simulink model "bbw"  (Simulink 8.7)
settings: Solver=FixedStepDiscrete  StartTime=0.0  StopTime=30  FixedStep=T_sim  RelTol=1e-6
PostLoadFcn:
  | parameters
undefined symbols (not defined in the file): distrib, Fc_table_x, Fc_table_y, I, M, maxBrakeTorque, R, slip_abs_on, T_abs, T_brake_ctrl, T_brake_pedal, T_spd_est, T_veh, use_division, v0, v_max, w0, w_max
settings Model: Creator=yt59680  LastModifiedBy=pfj01
settings SolverCC: AutoInsertRateTranBlk=on
settings DataIOCC: SignalLoggingSaveFormat=ModelDataLogs
settings OptimizationCC: ExpressionDepthLimit=2147483647
settings DebuggingCC: SolverPrmCheckMsg=warning  InvalidFcnCallConnMsg=warning  FcnCallInpInsideContextMsg=UseLocalSettings  AllowSymbolicDim=off  StateNameClashWarn=warning  StrictBusMsg=Warning
settings HardwareCC: TargetBitPerPointer=64  TargetLongLongMode=on  TargetIntDivRoundTo=Zero  TargetEndianess=LittleEndian  TargetWordSize=64  TargetHWDeviceType=MATLAB Host  ProdEqTarget=off
settings RTWCC: SystemTargetFile=rsim.tlc  TemplateMakefile=rsim_default_tmf  Description=Rapid Simulation Target
settings TargetCC: ParMdlRefBuildCompliant=on  ConcurrentExecutionCompliant=on  MatFileLogging=on
settings CustomProperty: DataType=string  Value=Auto

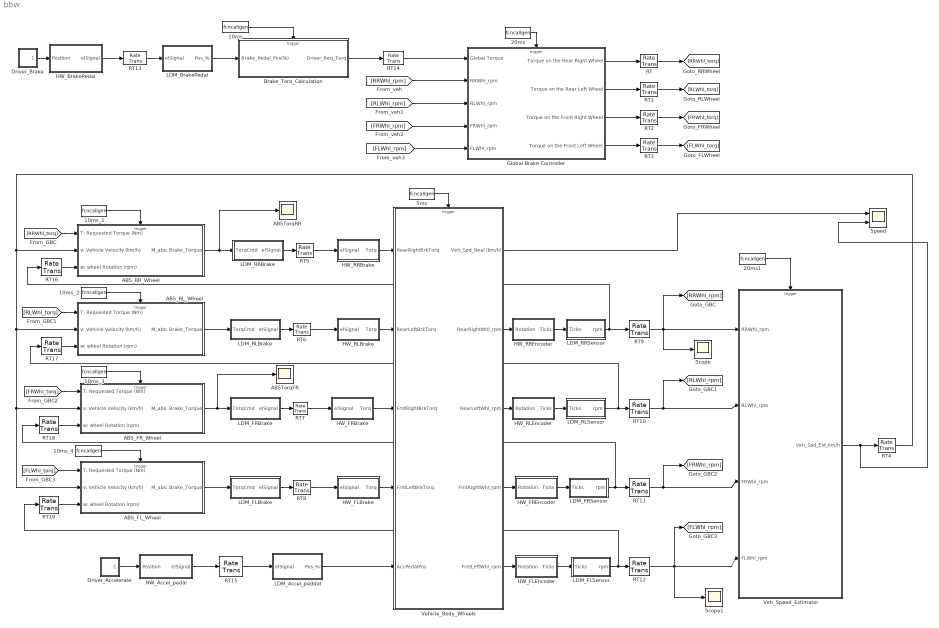
== system bbw ==
  10ms : S-Function  FunctionName=fcncallgen  Parameters=sample_time,numberOfIterations  SFunctionDeploymentMode=off  EnableBusSupport=off  mask(Function-Call Generator){sample_time=T_brake_pedal, numberOfIterations=1}
      mask prompts: sample_time "Simulink:masks:SampleTime_MP"; numberOfIterations "Simulink:masks:NumberOfIterations_MP"
      mask help: Simulink:masks:FunctionCallGenerator_MD
      mask init:
      | if ~isempty(numberOfIterations) & length(numberOfIterations) == 1 & (numberOfIterations > 1),
      | str=sprintf('iterate I = 1:%d',numberOfIterations);
      | else, str = 'f()';
      | end;
      mask Help: This block executes a function-call subsystem at the rate specified by the sample time and a specified number of times.
      mask Display: disp(str)
  10ms_1 : S-Function  FunctionName=fcncallgen  Parameters=sample_time,numberOfIterations  SFunctionDeploymentMode=off  EnableBusSupport=off  mask(Function-Call Generator){sample_time=T_abs, numberOfIterations=1}
      mask prompts: sample_time "Simulink:masks:SampleTime_MP"; numberOfIterations "Simulink:masks:NumberOfIterations_MP"
      mask help: Simulink:masks:FunctionCallGenerator_MD
      mask init:
      | if ~isempty(numberOfIterations) & length(numberOfIterations) == 1 & (numberOfIterations > 1),
      | str=sprintf('iterate I = 1:%d',numberOfIterations);
      | else, str = 'f()';
      | end;
      mask Help: This block executes a function-call subsystem at the rate specified by the sample time and a specified number of times.
      mask Display: disp(str)
  10ms_2 : S-Function  FunctionName=fcncallgen  Parameters=sample_time,numberOfIterations  SFunctionDeploymentMode=off  EnableBusSupport=off  mask(Function-Call Generator){sample_time=T_abs, numberOfIterations=1}
      mask prompts: sample_time "Simulink:masks:SampleTime_MP"; numberOfIterations "Simulink:masks:NumberOfIterations_MP"
      mask help: Simulink:masks:FunctionCallGenerator_MD
      mask init:
      | if ~isempty(numberOfIterations) & length(numberOfIterations) == 1 & (numberOfIterations > 1),
      | str=sprintf('iterate I = 1:%d',numberOfIterations);
      | else, str = 'f()';
      | end;
      mask Help: This block executes a function-call subsystem at the rate specified by the sample time and a specified number of times.
      mask Display: disp(str)
  10ms_3 : S-Function  FunctionName=fcncallgen  Parameters=sample_time,numberOfIterations  SFunctionDeploymentMode=off  EnableBusSupport=off  mask(Function-Call Generator){sample_time=T_abs, numberOfIterations=1}
      mask prompts: sample_time "Simulink:masks:SampleTime_MP"; numberOfIterations "Simulink:masks:NumberOfIterations_MP"
      mask help: Simulink:masks:FunctionCallGenerator_MD
      mask init:
      | if ~isempty(numberOfIterations) & length(numberOfIterations) == 1 & (numberOfIterations > 1),
      | str=sprintf('iterate I = 1:%d',numberOfIterations);
      | else, str = 'f()';
      | end;
      mask Help: This block executes a function-call subsystem at the rate specified by the sample time and a specified number of times.
      mask Display: disp(str)
  10ms_4 : S-Function  FunctionName=fcncallgen  Parameters=sample_time,numberOfIterations  SFunctionDeploymentMode=off  EnableBusSupport=off  mask(Function-Call Generator){sample_time=T_abs, numberOfIterations=1}
      mask prompts: sample_time "Simulink:masks:SampleTime_MP"; numberOfIterations "Simulink:masks:NumberOfIterations_MP"
      mask help: Simulink:masks:FunctionCallGenerator_MD
      mask init:
      | if ~isempty(numberOfIterations) & length(numberOfIterations) == 1 & (numberOfIterations > 1),
      | str=sprintf('iterate I = 1:%d',numberOfIterations);
      | else, str = 'f()';
      | end;
      mask Help: This block executes a function-call subsystem at the rate specified by the sample time and a specified number of times.
      mask Display: disp(str)
  20ms : S-Function  FunctionName=fcncallgen  Parameters=sample_time,numberOfIterations  SFunctionDeploymentMode=off  EnableBusSupport=off  mask(Function-Call Generator){sample_time=T_brake_ctrl, numberOfIterations=1}
      mask prompts: sample_time "Simulink:masks:SampleTime_MP"; numberOfIterations "Simulink:masks:NumberOfIterations_MP"
      mask help: Simulink:masks:FunctionCallGenerator_MD
      mask init:
      | if ~isempty(numberOfIterations) & length(numberOfIterations) == 1 & (numberOfIterations > 1),
      | str=sprintf('iterate I = 1:%d',numberOfIterations);
      | else, str = 'f()';
      | end;
      mask Help: This block executes a function-call subsystem at the rate specified by the sample time and a specified number of times.
      mask Display: disp(str)
  20ms1 : S-Function  FunctionName=fcncallgen  Parameters=sample_time,numberOfIterations  SFunctionDeploymentMode=off  EnableBusSupport=off  mask(Function-Call Generator){sample_time=T_spd_est, numberOfIterations=1}
      mask prompts: sample_time "Simulink:masks:SampleTime_MP"; numberOfIterations "Simulink:masks:NumberOfIterations_MP"
      mask help: Simulink:masks:FunctionCallGenerator_MD
      mask init:
      | if ~isempty(numberOfIterations) & length(numberOfIterations) == 1 & (numberOfIterations > 1),
      | str=sprintf('iterate I = 1:%d',numberOfIterations);
      | else, str = 'f()';
      | end;
      mask Help: This block executes a function-call subsystem at the rate specified by the sample time and a specified number of times.
      mask Display: disp(str)
  5ms : S-Function  FunctionName=fcncallgen  Parameters=sample_time,numberOfIterations  SFunctionDeploymentMode=off  EnableBusSupport=off  mask(Function-Call Generator){sample_time=T_veh, numberOfIterations=1}
      mask prompts: sample_time "Simulink:masks:SampleTime_MP"; numberOfIterations "Simulink:masks:NumberOfIterations_MP"
      mask help: Simulink:masks:FunctionCallGenerator_MD
      mask init:
      | if ~isempty(numberOfIterations) & length(numberOfIterations) == 1 & (numberOfIterations > 1),
      | str=sprintf('iterate I = 1:%d',numberOfIterations);
      | else, str = 'f()';
      | end;
      mask Help: This block executes a function-call subsystem at the rate specified by the sample time and a specified number of times.
      mask Display: disp(str)
  ABSTorqFR : Scope
  ABSTorqRR : Scope
  ABS_FL_Wheel : Subsystem  TreatAsAtomicUnit=on
  ABS_FR_Wheel : Subsystem  TreatAsAtomicUnit=on
  ABS_RL_Wheel : Subsystem  TreatAsAtomicUnit=on
  ABS_RR_Wheel : Subsystem  TreatAsAtomicUnit=on
  Brake_Torq_Calculation : Subsystem  TreatAsAtomicUnit=on
  Driver_Accelerate : Subsystem  mask(Repeating table){rep_seq_t=[0 1 10.5 11 100], rep_seq_y=[0 100 100 0 0]}
      mask prompts: rep_seq_t "Simulink:masks:TimeValues_MP"; rep_seq_y "Simulink:masks:OutputValues_MP"
      mask help: Simulink:masks:RepeatingTable_MD
      mask init:
      | X = [];
      | Y = [];
      | if (length(rep_seq_t) ~= length(rep_seq_y)),
      |   error('Length of time vector and output vector must be the same.')
      | end
      | dbl_rep_seq_t = double(rep_seq_t);
      | dbl_rep_seq_y = double(rep_seq_y);
      | period = max(dbl_rep_seq_t) - min(dbl_rep_seq_t);
      | period = slResolve(sprintf('%0.5g',period), gcbh);
      | [X, Y] = genRepeatingSequenceBlockIconData(dbl_rep_seq_t, dbl_rep_seq_y);
      mask Help: Repeats cycle given in table. Time values should be monotonically increasing.
      mask Display: plot(X, Y )
  Driver_Brake : Subsystem  mask(Repeating table){rep_seq_t=[0 19.5 20 100], rep_seq_y=[0 0 100 100]}
      mask prompts: rep_seq_t "Simulink:masks:TimeValues_MP"; rep_seq_y "Simulink:masks:OutputValues_MP"
      mask help: Simulink:masks:RepeatingTable_MD
      mask init: same as bbw/Driver_Accelerate
      mask Help: Repeats cycle given in table. Time values should be monotonically increasing.
      mask Display: plot(X, Y )
  Global Brake Controller : Subsystem  TreatAsAtomicUnit=on
  HW_Accel_pedal : Subsystem
  HW_BrakePedal : Subsystem
  HW_FLBrake : Subsystem
  HW_FLEncoder : Subsystem
  HW_FRBrake : Subsystem
  HW_FREncoder : Subsystem
  HW_RLBrake : Subsystem
  HW_RLEncoder : Subsystem
  HW_RRBrake : Subsystem
  HW_RREncoder : Subsystem
  LDM_Accel_peddal : Subsystem
  LDM_BrakePedal : Subsystem
  LDM_FLBrake : Subsystem
  LDM_FLSensor : Subsystem
  LDM_FRBrake : Subsystem
  LDM_FRSensor : Subsystem
  LDM_RLBrake : Subsystem
  LDM_RLSensor : Subsystem
  LDM_RRBrake : Subsystem
  LDM_RRSensor : Subsystem
  RT{,1..3,5..8,13..15} (11 alike) : RateTransition
  RT{9..12,16..19} (8 alike) : RateTransition  X0=w0*30/pi
  RT4 : RateTransition  X0=v0*3.6
  Scope : Scope
  Scope1 : Scope
  Speed : Scope  NumInputPorts=2
  Veh_Speed_Estimator : Subsystem  TreatAsAtomicUnit=on
  Vehicle_Body_Wheels : Subsystem
  wires:
  10ms/1 -> Brake_Torq_Calculation/Trigger
  20ms/1 -> Global Brake Controller/Trigger
  Global Brake Controller/1(Torque on the Rear Right Wheel) -> RT/1
  Global Brake Controller/2(Torque on the Rear Left Wheel) -> RT1/1
  Global Brake Controller/3(Torque on the Front Right Wheel) -> RT2/1
  10ms_1/1 -> ABS_RR_Wheel/Trigger
  ABS_RR_Wheel/1(M_abs: Brake_Torque) -> ABSTorqRR/1, LDM_RRBrake/1(TorqCmd)
  RT5/1 -> HW_RRBrake/1(elSignal)
  Vehicle_Body_Wheels/2(RearRightWhl_rpm) -> HW_RREncoder/1(Rotation)
  Global Brake Controller/4(Torque on the Front Left Wheel) -> RT3/1
  [RRWhl_torq] -> ABS_RR_Wheel/1(T: Requested Torque (Nm))
  ABS_RL_Wheel/1(M_abs: Brake_Torque) -> LDM_RLBrake/1(TorqCmd)
  RT6/1 -> HW_RLBrake/1(elSignal)
  Vehicle_Body_Wheels/3(RearLeftWhl_rpm) -> HW_RLEncoder/1(Rotation)
  [RLWhl_torq] -> ABS_RL_Wheel/1(T: Requested Torque (Nm))
  ABS_FR_Wheel/1(M_abs: Brake_Torque) -> ABSTorqFR/1, LDM_FRBrake/1(TorqCmd)
  RT7/1 -> HW_FRBrake/1(elSignal)
  Vehicle_Body_Wheels/4(FrntRightWhl_rpm) -> HW_FREncoder/1(Rotation)
  [FRWhl_torq] -> ABS_FR_Wheel/1(T: Requested Torque (Nm))
  ABS_FL_Wheel/1(M_abs: Brake_Torque) -> LDM_FLBrake/1(TorqCmd)
  RT8/1 -> HW_FLBrake/1(elSignal)
  Vehicle_Body_Wheels/5(FrntLeftWhl_rpm) -> HW_FLEncoder/1(Rotation)
  [FLWhl_torq] -> ABS_FL_Wheel/1(T: Requested Torque (Nm))
  Driver_Brake/1(Out1) -> HW_BrakePedal/1(Position)
  Brake_Torq_Calculation/1(Driver_Req_Torq) -> RT14/1
  RT14/1 -> Global Brake Controller/1(Global Torque)
  [RRWhl_rpm] -> Global Brake Controller/2(RRWhl_rpm)
  [RLWhl_rpm] -> Global Brake Controller/3(RLWhl_rpm)
  [FRWhl_rpm] -> Global Brake Controller/4(FRWhl_rpm)
  [FLWhl_rpm] -> Global Brake Controller/5(FLWhl_rpm)
  RT/1 -> [RRWhl_torq]
  RT1/1 -> [RLWhl_torq]
  RT2/1 -> [FRWhl_torq]
  RT3/1 -> [FLWhl_torq]
  RT4/1 -> ABS_FR_Wheel/2(v: Vehicle Velocity (km/h)), ABS_FL_Wheel/2(v: Vehicle Velocity (km/h)), ABS_RL_Wheel/2(v: Vehicle Velocity (km/h)), ABS_RR_Wheel/2(v: Vehicle Velocity (km/h))
  LDM_RRBrake/1(elSignal) -> RT5/1
  HW_RRBrake/1(Torq) -> Vehicle_Body_Wheels/1(RearRightBrkTorq)
  LDM_RLBrake/1(elSignal) -> RT6/1
  HW_RLBrake/1(Torq) -> Vehicle_Body_Wheels/2(RearLeftBrkTorq)
  LDM_FRBrake/1(elSignal) -> RT7/1
  HW_FRBrake/1(Torq) -> Vehicle_Body_Wheels/3(FrntRightBrkTorq)
  LDM_FLBrake/1(elSignal) -> RT8/1
  HW_FLBrake/1(Torq) -> Vehicle_Body_Wheels/4(FrntLeftBrkTorq)
  HW_RREncoder/1(Ticks) -> LDM_RRSensor/1(Ticks)
  HW_RLEncoder/1(Ticks) -> LDM_RLSensor/1(Ticks)
  HW_FREncoder/1(Ticks) -> LDM_FRSensor/1(Ticks)
  LDM_RRSensor/1(rpm) -> RT16/1, RT9/1
  LDM_RLSensor/1(rpm) -> RT10/1, RT17/1
  LDM_FRSensor/1(rpm) -> RT11/1, RT18/1
  HW_BrakePedal/1(elSignal) -> RT13/1
  LDM_BrakePedal/1(Pos_%) -> Brake_Torq_Calculation/1(Brake_Pedal_Pos(%))
  Driver_Accelerate/1(Out1) -> HW_Accel_pedal/1(Position)
  5ms/1 -> Vehicle_Body_Wheels/Trigger
  10ms_2/1 -> ABS_RL_Wheel/Trigger
  10ms_3/1 -> ABS_FR_Wheel/Trigger
  10ms_4/1 -> ABS_FL_Wheel/Trigger
  20ms1/1 -> Veh_Speed_Estimator/Trigger
  Veh_Speed_Estimator/1(Veh_Spd_Est_km/h) -> RT4/1, Speed/2
  Vehicle_Body_Wheels/1(Veh_Spd_Real (km/h)) -> Speed/1
  RT13/1 -> LDM_BrakePedal/1(elSignal)
  HW_Accel_pedal/1(elSignal) -> RT15/1
  LDM_Accel_peddal/1(Pos_%) -> Vehicle_Body_Wheels/5(AccPedalPos)
  RT15/1 -> LDM_Accel_peddal/1(elSignal)
  LDM_FLSensor/1(rpm) -> RT19/1, RT12/1
  RT16/1 -> ABS_RR_Wheel/3(w: wheel Rotation (rpm))
  RT17/1 -> ABS_RL_Wheel/3(w: wheel Rotation (rpm))
  RT18/1 -> ABS_FR_Wheel/3(w: wheel Rotation (rpm))
  RT19/1 -> ABS_FL_Wheel/3(w: wheel Rotation (rpm))
  RT9/1 -> Veh_Speed_Estimator/1(RRWhl_rpm), [RRWhl_rpm], Scope/1
  RT10/1 -> Veh_Speed_Estimator/2(RLWhl_rpm), [RLWhl_rpm]
  RT11/1 -> Veh_Speed_Estimator/3(FRWhl_rpm), [FRWhl_rpm]
  HW_FLEncoder/1(Ticks) -> LDM_FLSensor/1(Ticks)
  RT12/1 -> [FLWhl_rpm], Veh_Speed_Estimator/4(FLWhl_rpm), Scope1/1

== system bbw/ABS_FL_Wheel ==
  T: Requested Torque (Nm) : Inport
  v: Vehicle Velocity (km/h) : Inport  Port=2
  w: wheel Rotation (rpm) : Inport  Port=3
  function : TriggerPort  TriggerType=function-call  VariantControl=Variant
  If v>=10 km/h : Subsystem  TreatAsAtomicUnit=on
  Threshold_10km/h : Switch  Threshold=10
  M_abs: Brake_Torque : Outport
  wires:
  v: Vehicle Velocity (km/h)/1 -> Threshold_10km/h/2, If v>=10 km/h/2(v_km/h)
  T: Requested Torque (Nm)/1 -> Threshold_10km/h/3, If v>=10 km/h/1(T_Nm)
  If v>=10 km/h/1(BrakeTorque) -> Threshold_10km/h/1
  Threshold_10km/h/1 -> M_abs: Brake_Torque/1
  w: wheel Rotation (rpm)/1 -> If v>=10 km/h/3(w_rpm)

== system bbw/ABS_FR_Wheel ==
  T: Requested Torque (Nm) : Inport
  v: Vehicle Velocity (km/h) : Inport  Port=2
  w: wheel Rotation (rpm) : Inport  Port=3
  function : TriggerPort  TriggerType=function-call  VariantControl=Variant
  If v>=10 km/h : Subsystem  TreatAsAtomicUnit=on
  Threshold_10km/h : Switch  Threshold=10
  M_abs: Brake_Torque : Outport
  wires:
  v: Vehicle Velocity (km/h)/1 -> Threshold_10km/h/2, If v>=10 km/h/2(v_km/h)
  T: Requested Torque (Nm)/1 -> Threshold_10km/h/3, If v>=10 km/h/1(T_Nm)
  If v>=10 km/h/1(BrakeTorque) -> Threshold_10km/h/1
  Threshold_10km/h/1 -> M_abs: Brake_Torque/1
  w: wheel Rotation (rpm)/1 -> If v>=10 km/h/3(w_rpm)

== system bbw/ABS_RL_Wheel ==
  T: Requested Torque (Nm) : Inport
  v: Vehicle Velocity (km/h) : Inport  Port=2
  w: wheel Rotation (rpm) : Inport  Port=3
  function : TriggerPort  TriggerType=function-call  VariantControl=Variant
  If v>=10 km/h : Subsystem  TreatAsAtomicUnit=on
  Threshold_10km/h : Switch  Threshold=10
  M_abs: Brake_Torque : Outport
  wires:
  v: Vehicle Velocity (km/h)/1 -> Threshold_10km/h/2, If v>=10 km/h/2(v_km/h)
  T: Requested Torque (Nm)/1 -> Threshold_10km/h/3, If v>=10 km/h/1(T_Nm)
  If v>=10 km/h/1(BrakeTorque) -> Threshold_10km/h/1
  Threshold_10km/h/1 -> M_abs: Brake_Torque/1
  w: wheel Rotation (rpm)/1 -> If v>=10 km/h/3(w_rpm)

== system bbw/ABS_RR_Wheel ==
  T: Requested Torque (Nm) : Inport
  v: Vehicle Velocity (km/h) : Inport  Port=2
  w: wheel Rotation (rpm) : Inport  Port=3
  function : TriggerPort  TriggerType=function-call  VariantControl=Variant
  If v>=10 km/h : Subsystem  TreatAsAtomicUnit=on
  Threshold_10km/h : Switch  Threshold=10
  M_abs: Brake_Torque : Outport
  wires:
  v: Vehicle Velocity (km/h)/1 -> Threshold_10km/h/2, If v>=10 km/h/2(v_km/h)
  T: Requested Torque (Nm)/1 -> Threshold_10km/h/3, If v>=10 km/h/1(T_Nm)
  If v>=10 km/h/1(BrakeTorque) -> Threshold_10km/h/1
  Threshold_10km/h/1 -> M_abs: Brake_Torque/1
  w: wheel Rotation (rpm)/1 -> If v>=10 km/h/3(w_rpm)

== system bbw/Brake_Torq_Calculation ==
  Brake_Pedal_Pos(%) : Inport
  function : TriggerPort  TriggerType=function-call  VariantControl=Variant
  Gain1 : Gain  Gain=maxBrakeTorque/100  OutMin=0  OutMax=4000
  Driver_Req_Torq : Outport
  wires:
  Gain1/1 -> Driver_Req_Torq/1
  Brake_Pedal_Pos(%)/1 -> Gain1/1

== system bbw/Driver_Accelerate ==
  Clock : Clock
      settings: DisableCoverage=on
  Constant : Constant  DisableCoverage=on  Value=period
  Look-Up Table1 : Lookup_n-D  DisableCoverage=on  NumberOfTableDimensions=1  BreakpointsForDimension1=rep_seq_t - min(rep_seq_t)  BreakpointsForDimension3=[5, 7]  Table=rep_seq_y  InternalRulePriority=Speed  SaturateOnIntegerOverflow=on  InputSameDT=on
  Math Function : Math  DisableCoverage=on  Operator=rem  SaturateOnIntegerOverflow=on
  Output : SignalConversion  OverrideOpt=off
  Sum : Sum  DisableCoverage=on  Inputs=+-  SaturateOnIntegerOverflow=on  InputSameDT=on  OutDataTypeStr=Inherit: Same as first input
  startTime : S-Function  DisableCoverage=on  FunctionName=sfun_tstart  SFunctionDeploymentMode=off  EnableBusSupport=off
  Out1 : Outport
  wires:
  Constant/1 -> Math Function/2
  Output/1 -> Out1/1
  Look-Up Table1/1 -> Output/1
  startTime/1 -> Sum/2
  Clock/1 -> Sum/1
  Sum/1 -> Math Function/1
  Math Function/1 -> Look-Up Table1/1

== system bbw/Driver_Brake ==
  Clock : Clock
      settings: DisableCoverage=on
  Constant : Constant  DisableCoverage=on  Value=period
  Look-Up Table1 : Lookup_n-D  DisableCoverage=on  NumberOfTableDimensions=1  BreakpointsForDimension1=rep_seq_t - min(rep_seq_t)  BreakpointsForDimension3=[5, 7]  Table=rep_seq_y  InternalRulePriority=Speed  SaturateOnIntegerOverflow=on  InputSameDT=on
  Math Function : Math  DisableCoverage=on  Operator=rem  SaturateOnIntegerOverflow=on
  Output : SignalConversion  OverrideOpt=off
  Sum : Sum  DisableCoverage=on  Inputs=+-  SaturateOnIntegerOverflow=on  InputSameDT=on  OutDataTypeStr=Inherit: Same as first input
  startTime : S-Function  DisableCoverage=on  FunctionName=sfun_tstart  SFunctionDeploymentMode=off  EnableBusSupport=off
  Out1 : Outport
  wires:
  Constant/1 -> Math Function/2
  Output/1 -> Out1/1
  Look-Up Table1/1 -> Output/1
  startTime/1 -> Sum/2
  Clock/1 -> Sum/1
  Sum/1 -> Math Function/1
  Math Function/1 -> Look-Up Table1/1

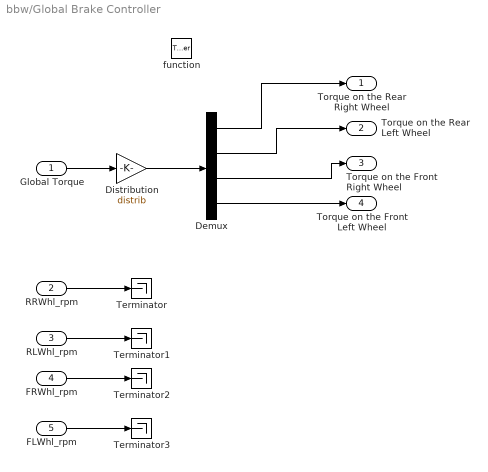
== system bbw/Global Brake Controller ==
  Global Torque : Inport
  RRWhl_rpm : Inport  Port=2
  RLWhl_rpm : Inport  Port=3
  FRWhl_rpm : Inport  Port=4
  FLWhl_rpm : Inport  Port=5
  function : TriggerPort  TriggerType=function-call  VariantControl=Variant
  Demux : Demux
  Distribution : Gain  Gain=distrib  OutMax=2000  OutDataTypeStr=double
  Terminator{,1..3} (4 alike) : Terminator
  Torque on the Rear Right Wheel : Outport
  Torque on the Rear Left Wheel : Outport  Port=2
  Torque on the Front Right Wheel : Outport  Port=3
  Torque on the Front Left Wheel : Outport  Port=4
  wires:
  Demux/3 -> Torque on the Front Right Wheel/1
  Demux/2 -> Torque on the Rear Left Wheel/1
  Demux/1 -> Torque on the Rear Right Wheel/1
  Demux/4 -> Torque on the Front Left Wheel/1
  Distribution/1 -> Demux/1
  Global Torque/1 -> Distribution/1
  RRWhl_rpm/1 -> Terminator/1
  RLWhl_rpm/1 -> Terminator1/1
  FRWhl_rpm/1 -> Terminator2/1
  FLWhl_rpm/1 -> Terminator3/1

== system bbw/HW_Accel_pedal ==
  Position : Inport
  Pedal_map : Saturate  UpperLimit=100  LowerLimit=0
  elSignal : Outport
  wires:
  Position/1 -> Pedal_map/1
  Pedal_map/1 -> elSignal/1

== system bbw/HW_BrakePedal ==
  Position : Inport
  Pedal_map : Saturate  UpperLimit=100  LowerLimit=0
  elSignal : Outport
  wires:
  Position/1 -> Pedal_map/1
  Pedal_map/1 -> elSignal/1

== system bbw/HW_FLBrake ==
  elSignal : Inport
  Torq : Outport
  wires:
  elSignal/1 -> Torq/1

== system bbw/HW_FLEncoder ==
  Rotation : Inport
  to_int1 : Rounding  Operator=round
  Ticks : Outport
  wires:
  Rotation/1 -> to_int1/1
  to_int1/1 -> Ticks/1

== system bbw/HW_FRBrake ==
  elSignal : Inport
  Torq : Outport
  wires:
  elSignal/1 -> Torq/1

== system bbw/HW_FREncoder ==
  Rotation : Inport
  to_int : Rounding  Operator=round
  Ticks : Outport
  wires:
  Rotation/1 -> to_int/1
  to_int/1 -> Ticks/1

== system bbw/HW_RLBrake ==
  elSignal : Inport
  Torq : Outport
  wires:
  elSignal/1 -> Torq/1

== system bbw/HW_RLEncoder ==
  Rotation : Inport
  to_int : Rounding  Operator=round
  Ticks : Outport
  wires:
  Rotation/1 -> to_int/1
  to_int/1 -> Ticks/1

== system bbw/HW_RRBrake ==
  elSignal : Inport
  Torq : Outport
  wires:
  elSignal/1 -> Torq/1

== system bbw/HW_RREncoder ==
  Rotation : Inport
  to_int : Rounding  Operator=round
  Ticks : Outport
  wires:
  Rotation/1 -> to_int/1
  to_int/1 -> Ticks/1

== system bbw/LDM_Accel_peddal ==
  elSignal : Inport
  to_int : Rounding  Operator=round
  Pos_% : Outport
  wires:
  elSignal/1 -> to_int/1
  to_int/1 -> Pos_%/1

== system bbw/LDM_BrakePedal ==
  elSignal : Inport
  round_to_int : Rounding  Operator=round
  Pos_% : Outport
  wires:
  elSignal/1 -> round_to_int/1
  round_to_int/1 -> Pos_%/1

== system bbw/LDM_FLBrake ==
  TorqCmd : Inport
  elSignal : Outport
  wires:
  TorqCmd/1 -> elSignal/1

== system bbw/LDM_FLSensor ==
  Ticks : Inport
  rpm : Outport
  wires:
  Ticks/1 -> rpm/1

== system bbw/LDM_FRBrake ==
  TorqCmd : Inport
  elSignal : Outport
  wires:
  TorqCmd/1 -> elSignal/1

== system bbw/LDM_FRSensor ==
  Ticks : Inport
  rpm : Outport
  wires:
  Ticks/1 -> rpm/1

== system bbw/LDM_RLBrake ==
  TorqCmd : Inport
  elSignal : Outport
  wires:
  TorqCmd/1 -> elSignal/1

== system bbw/LDM_RLSensor ==
  Ticks : Inport
  rpm : Outport
  wires:
  Ticks/1 -> rpm/1

== system bbw/LDM_RRBrake ==
  TorqCmd : Inport
  elSignal : Outport
  wires:
  TorqCmd/1 -> elSignal/1

== system bbw/LDM_RRSensor ==
  Ticks : Inport
  rpm : Outport
  wires:
  Ticks/1 -> rpm/1

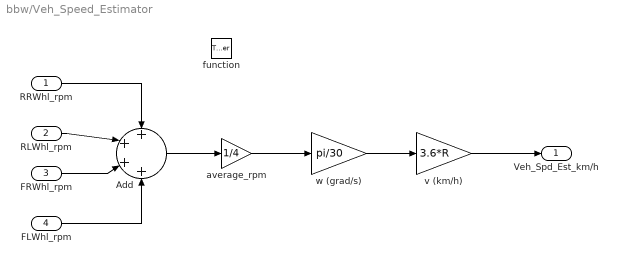
== system bbw/Veh_Speed_Estimator ==
  RRWhl_rpm : Inport
  RLWhl_rpm : Inport  Port=2
  FRWhl_rpm : Inport  Port=3
  FLWhl_rpm : Inport  Port=4
  function : TriggerPort  TriggerType=function-call  VariantControl=Variant
  Add : Sum  Inputs=++++
  average_rpm : Gain  Gain=1/4  OutMin=0  OutMax=2000  OutDataTypeStr=double
  v (km/h) : Gain  Gain=3.6*R  OutMin=0  OutMax=200
  w (grad/s) : Gain  Gain=pi/30  OutMin=0  OutMax=250
  Veh_Spd_Est_km/h : Outport
  wires:
  v (km/h)/1 -> Veh_Spd_Est_km/h/1
  average_rpm/1 -> w (grad/s)/1
  w (grad/s)/1 -> v (km/h)/1
  Add/1 -> average_rpm/1
  FLWhl_rpm/1 -> Add/4
  FRWhl_rpm/1 -> Add/3
  RLWhl_rpm/1 -> Add/2
  RRWhl_rpm/1 -> Add/1

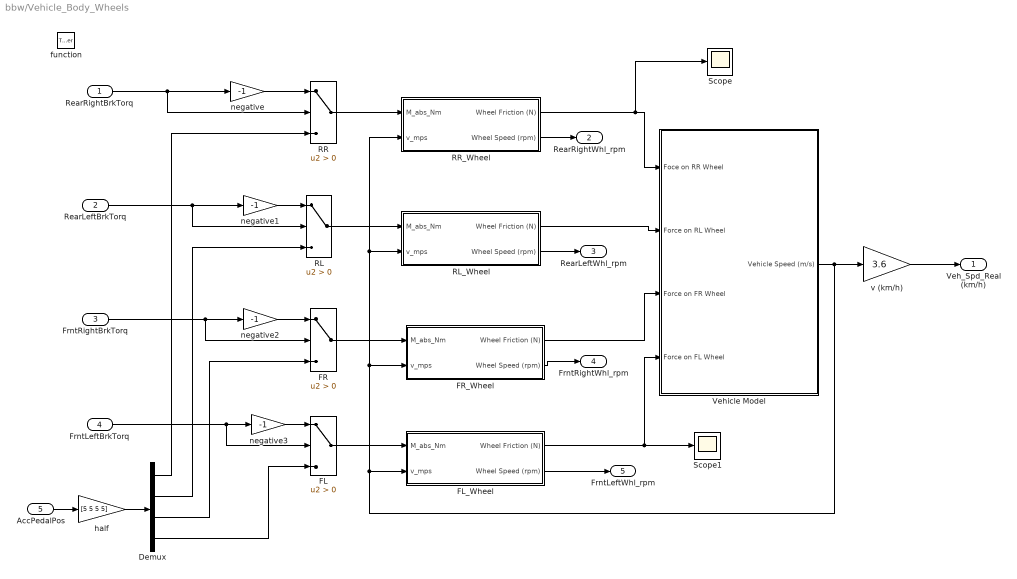
== system bbw/Vehicle_Body_Wheels ==
  RearRightBrkTorq : Inport
  RearLeftBrkTorq : Inport  Port=2
  FrntRightBrkTorq : Inport  Port=3
  FrntLeftBrkTorq : Inport  Port=4
  AccPedalPos : Inport  Port=5
  function : TriggerPort  TriggerType=function-call  VariantControl=Variant
  Demux : Demux
  FL : Switch  Criteria=u2 > Threshold
  FL_Wheel : Subsystem  TreatAsAtomicUnit=on
  FR : Switch  Criteria=u2 > Threshold
  FR_Wheel : Subsystem  TreatAsAtomicUnit=on
  RL : Switch  Criteria=u2 > Threshold
  RL_Wheel : Subsystem  TreatAsAtomicUnit=on
  RR : Switch  Criteria=u2 > Threshold
  RR_Wheel : Subsystem  TreatAsAtomicUnit=on
  Scope : Scope
  Scope1 : Scope
  Vehicle Model : Subsystem  TreatAsAtomicUnit=on
      settings: MinAlgLoopOccurrences=on
  half : Gain  Gain=[5 5 5 5]  ParamDataTypeStr=double
  negative{,1..3} (4 alike) : Gain  Gain=-1
  v (km/h) : Gain  Gain=3.6  OutMin=0  OutMax=200
  Veh_Spd_Real (km/h) : Outport
  RearRightWhl_rpm : Outport  Port=2
  RearLeftWhl_rpm : Outport  Port=3
  FrntRightWhl_rpm : Outport  Port=4
  FrntLeftWhl_rpm : Outport  Port=5
  wires:
  Vehicle Model/1(Vehicle Speed (m/s)) -> v (km/h)/1, RR_Wheel/2(v_mps), RL_Wheel/2(v_mps), FR_Wheel/2(v_mps), FL_Wheel/2(v_mps)
  RR_Wheel/2(Wheel Speed (rpm)) -> RearRightWhl_rpm/1
  RR_Wheel/1(Wheel Friction (N)) -> Scope/1, Vehicle Model/1(Foce on RR Wheel)
  RL_Wheel/2(Wheel Speed (rpm)) -> RearLeftWhl_rpm/1
  RL_Wheel/1(Wheel Friction (N)) -> Vehicle Model/2(Force on RL Wheel)
  FR_Wheel/2(Wheel Speed (rpm)) -> FrntRightWhl_rpm/1
  FR_Wheel/1(Wheel Friction (N)) -> Vehicle Model/3(Force on FR Wheel)
  FL_Wheel/1(Wheel Friction (N)) -> Scope1/1, Vehicle Model/4(Force on FL Wheel)
  AccPedalPos/1 -> half/1
  FR/1 -> FR_Wheel/1(M_abs_Nm)
  FrntRightBrkTorq/1 -> FR/2, negative2/1
  FL/1 -> FL_Wheel/1(M_abs_Nm)
  FrntLeftBrkTorq/1 -> FL/2, negative3/1
  RR/1 -> RR_Wheel/1(M_abs_Nm)
  RearRightBrkTorq/1 -> RR/2, negative/1
  RL/1 -> RL_Wheel/1(M_abs_Nm)
  RearLeftBrkTorq/1 -> RL/2, negative1/1
  half/1 -> Demux/1
  Demux/1 -> RR/3
  Demux/2 -> RL/3
  Demux/3 -> FR/3
  Demux/4 -> FL/3
  v (km/h)/1 -> Veh_Spd_Real (km/h)/1
  negative/1 -> RR/1
  negative1/1 -> RL/1
  negative2/1 -> FR/1
  negative3/1 -> FL/1
  FL_Wheel/2(Wheel Speed (rpm)) -> FrntLeftWhl_rpm/1

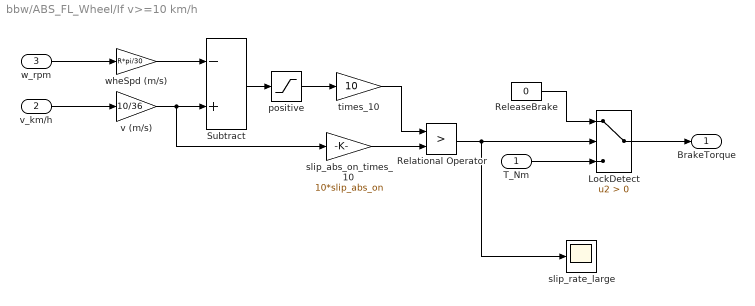
== system bbw/ABS_FL_Wheel/If v>=10 km/h ==
  T_Nm : Inport
  v_km/h : Inport  Port=2
  w_rpm : Inport  Port=3
  LockDetect : Switch  Criteria=u2 > Threshold
  Relational Operator : RelationalOperator  Operator=>  OutDataTypeStr=boolean
  ReleaseBrake : Constant  Value=0  OutDataTypeStr=uint8
  Subtract : Sum  Inputs=-+
  positive : Saturate  UpperLimit=inf  LowerLimit=0
  slip_abs_on_times_10 : Gain  Gain=10*slip_abs_on
  slip_rate_large : Scope
  times_10 : Gain  Gain=10
  v (m/s) : Gain  Gain=10/36  OutMin=0  OutMax=100
  wheSpd (m/s) : Gain  Gain=R*pi/30  OutMin=0  OutMax=100
  BrakeTorque : Outport
  wires:
  v (m/s)/1 -> Subtract/2, slip_abs_on_times_10/1
  wheSpd (m/s)/1 -> Subtract/1
  T_Nm/1 -> LockDetect/3
  ReleaseBrake/1 -> LockDetect/1
  LockDetect/1 -> BrakeTorque/1
  Relational Operator/1 -> LockDetect/2, slip_rate_large/1
  times_10/1 -> Relational Operator/1
  Subtract/1 -> positive/1
  v_km/h/1 -> v (m/s)/1
  w_rpm/1 -> wheSpd (m/s)/1
  slip_abs_on_times_10/1 -> Relational Operator/2
  positive/1 -> times_10/1

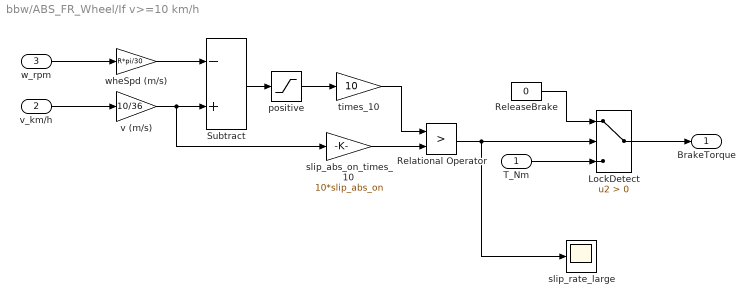
== system bbw/ABS_FR_Wheel/If v>=10 km/h ==
  T_Nm : Inport
  v_km/h : Inport  Port=2
  w_rpm : Inport  Port=3
  LockDetect : Switch  Criteria=u2 > Threshold
  Relational Operator : RelationalOperator  Operator=>  OutDataTypeStr=boolean
  ReleaseBrake : Constant  Value=0  OutDataTypeStr=uint8
  Subtract : Sum  Inputs=-+
  positive : Saturate  UpperLimit=inf  LowerLimit=0
  slip_abs_on_times_10 : Gain  Gain=10*slip_abs_on
  slip_rate_large : Scope
  times_10 : Gain  Gain=10
  v (m/s) : Gain  Gain=10/36  OutMin=0  OutMax=100
  wheSpd (m/s) : Gain  Gain=R*pi/30  OutMin=0  OutMax=100
  BrakeTorque : Outport
  wires:
  v (m/s)/1 -> Subtract/2, slip_abs_on_times_10/1
  wheSpd (m/s)/1 -> Subtract/1
  T_Nm/1 -> LockDetect/3
  ReleaseBrake/1 -> LockDetect/1
  LockDetect/1 -> BrakeTorque/1
  Relational Operator/1 -> LockDetect/2, slip_rate_large/1
  times_10/1 -> Relational Operator/1
  Subtract/1 -> positive/1
  v_km/h/1 -> v (m/s)/1
  w_rpm/1 -> wheSpd (m/s)/1
  slip_abs_on_times_10/1 -> Relational Operator/2
  positive/1 -> times_10/1

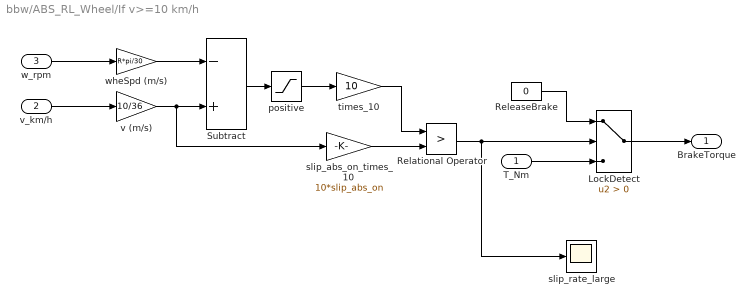
== system bbw/ABS_RL_Wheel/If v>=10 km/h ==
  T_Nm : Inport
  v_km/h : Inport  Port=2
  w_rpm : Inport  Port=3
  LockDetect : Switch  Criteria=u2 > Threshold
  Relational Operator : RelationalOperator  Operator=>  OutDataTypeStr=boolean
  ReleaseBrake : Constant  Value=0  OutDataTypeStr=uint8
  Subtract : Sum  Inputs=-+
  positive : Saturate  UpperLimit=inf  LowerLimit=0
  slip_abs_on_times_10 : Gain  Gain=10*slip_abs_on
  slip_rate_large : Scope
  times_10 : Gain  Gain=10
  v (m/s) : Gain  Gain=10/36  OutMin=0  OutMax=100
  wheSpd (m/s) : Gain  Gain=R*pi/30  OutMin=0  OutMax=100
  BrakeTorque : Outport
  wires:
  v (m/s)/1 -> Subtract/2, slip_abs_on_times_10/1
  wheSpd (m/s)/1 -> Subtract/1
  T_Nm/1 -> LockDetect/3
  ReleaseBrake/1 -> LockDetect/1
  LockDetect/1 -> BrakeTorque/1
  Relational Operator/1 -> LockDetect/2, slip_rate_large/1
  times_10/1 -> Relational Operator/1
  Subtract/1 -> positive/1
  v_km/h/1 -> v (m/s)/1
  w_rpm/1 -> wheSpd (m/s)/1
  slip_abs_on_times_10/1 -> Relational Operator/2
  positive/1 -> times_10/1

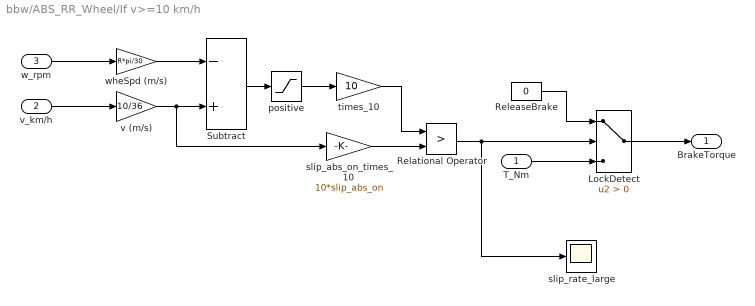
== system bbw/ABS_RR_Wheel/If v>=10 km/h ==
  T_Nm : Inport
  v_km/h : Inport  Port=2
  w_rpm : Inport  Port=3
  LockDetect : Switch  Criteria=u2 > Threshold
  Relational Operator : RelationalOperator  Operator=>  OutDataTypeStr=boolean
  ReleaseBrake : Constant  Value=0  OutDataTypeStr=uint8
  Subtract : Sum  Inputs=-+
  positive : Saturate  UpperLimit=inf  LowerLimit=0
  slip_abs_on_times_10 : Gain  Gain=10*slip_abs_on
  slip_rate_large : Scope
  times_10 : Gain  Gain=10
  v (m/s) : Gain  Gain=10/36  OutMin=0  OutMax=100
  wheSpd (m/s) : Gain  Gain=R*pi/30  OutMin=0  OutMax=100
  BrakeTorque : Outport
  wires:
  v (m/s)/1 -> Subtract/2, slip_abs_on_times_10/1
  wheSpd (m/s)/1 -> Subtract/1
  T_Nm/1 -> LockDetect/3
  ReleaseBrake/1 -> LockDetect/1
  LockDetect/1 -> BrakeTorque/1
  Relational Operator/1 -> LockDetect/2, slip_rate_large/1
  times_10/1 -> Relational Operator/1
  Subtract/1 -> positive/1
  v_km/h/1 -> v (m/s)/1
  w_rpm/1 -> wheSpd (m/s)/1
  slip_abs_on_times_10/1 -> Relational Operator/2
  positive/1 -> times_10/1

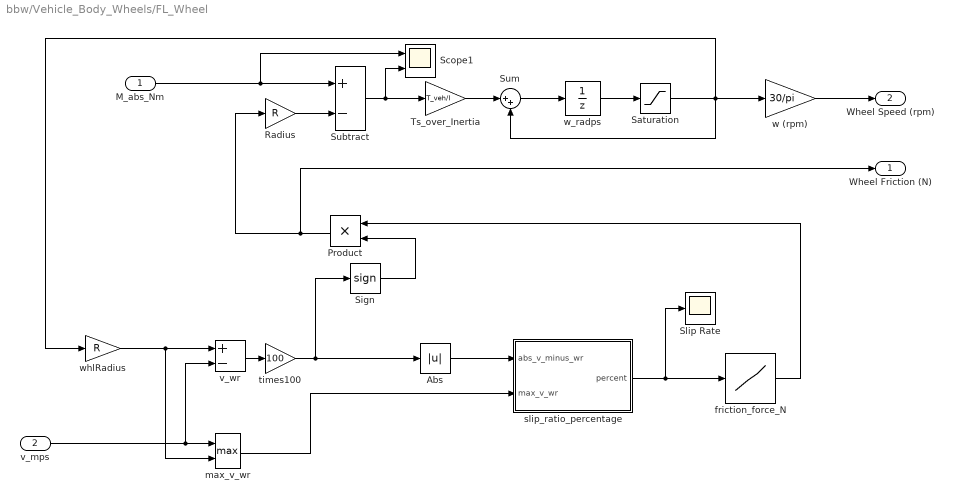
== system bbw/Vehicle_Body_Wheels/FL_Wheel ==
  M_abs_Nm : Inport
  v_mps : Inport  Port=2
  Abs : Abs
  Product : Product  RndMeth=Zero
  Radius : Gain  Gain=R
  Saturation : Saturate  UpperLimit=w_max  LowerLimit=0
  Scope1 : Scope  NumInputPorts=2
  Sign : Signum
  Slip Rate : Scope
  Subtract : Sum  Inputs=+-
  Sum : Sum  Inputs=|++
  Ts_over_Inertia : Gain  Gain=T_veh/I
  friction_force_N : Lookup  InputValues=Fc_table_x  Table=Fc_table_y  LookUpMeth=Interpolation-Use End Values  OutMin=0  OutMax=1000000  OutDataTypeStr=Inherit: Inherit via back propagation
  max_v_wr : MinMax  Function=max  Inputs=2
  slip_ratio_percentage : Subsystem
  times100 : Gain  Gain=100
  v_wr : Sum  Inputs=+-
  w (rpm) : Gain  Gain=30/pi  OutMin=0  OutMax=w_max*30/pi
  w_radps : UnitDelay  InitialCondition=w0  SampleTime=-1
  whlRadius : Gain  Gain=R  OutMin=0  OutMax=w_max/2
  Wheel Friction (N) : Outport
  Wheel Speed (rpm) : Outport  Port=2
  wires:
  M_abs_Nm/1 -> Subtract/1, Scope1/1
  v_mps/1 -> max_v_wr/1, v_wr/2
  w (rpm)/1 -> Wheel Speed (rpm)/1
  w_radps/1 -> Saturation/1
  Ts_over_Inertia/1 -> Sum/1
  Subtract/1 -> Ts_over_Inertia/1, Scope1/2
  Radius/1 -> Subtract/2
  Sign/1 -> Product/2
  max_v_wr/1 -> slip_ratio_percentage/2(max_v_wr)
  Product/1 -> Radius/1, Wheel Friction (N)/1
  v_wr/1 -> times100/1
  Abs/1 -> slip_ratio_percentage/1(abs_v_minus_wr)
  whlRadius/1 -> v_wr/1, max_v_wr/2
  slip_ratio_percentage/1(percent) -> friction_force_N/1, Slip Rate/1
  friction_force_N/1 -> Product/1
  Sum/1 -> w_radps/1
  Saturation/1 -> w (rpm)/1, whlRadius/1, Sum/2
  times100/1 -> Sign/1, Abs/1

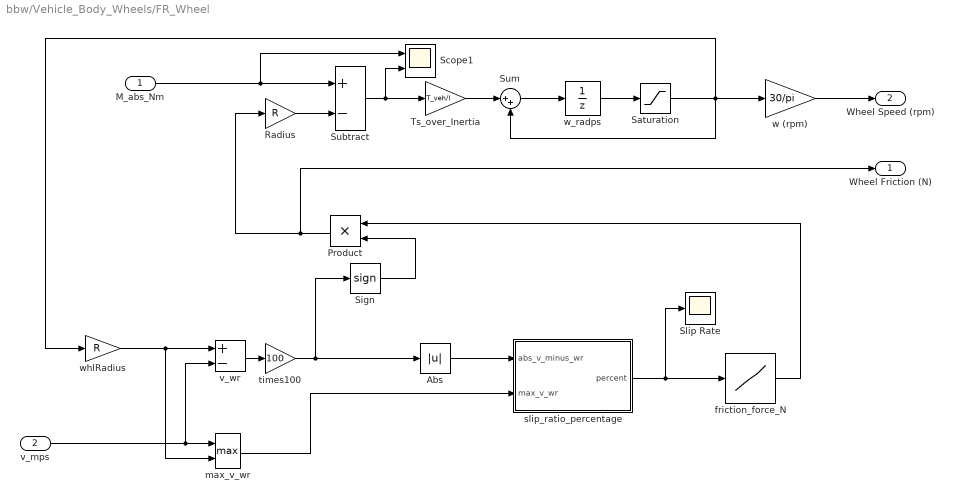
== system bbw/Vehicle_Body_Wheels/FR_Wheel ==
  M_abs_Nm : Inport
  v_mps : Inport  Port=2
  Abs : Abs
  Product : Product  RndMeth=Zero
  Radius : Gain  Gain=R
  Saturation : Saturate  UpperLimit=w_max  LowerLimit=0
  Scope1 : Scope  NumInputPorts=2
  Sign : Signum
  Slip Rate : Scope
  Subtract : Sum  Inputs=+-
  Sum : Sum  Inputs=|++
  Ts_over_Inertia : Gain  Gain=T_veh/I
  friction_force_N : Lookup  InputValues=Fc_table_x  Table=Fc_table_y  LookUpMeth=Interpolation-Use End Values  OutMin=0  OutMax=1000000  OutDataTypeStr=Inherit: Inherit via back propagation
  max_v_wr : MinMax  Function=max  Inputs=2
  slip_ratio_percentage : Subsystem
  times100 : Gain  Gain=100
  v_wr : Sum  Inputs=+-
  w (rpm) : Gain  Gain=30/pi  OutMin=0  OutMax=w_max*30/pi
  w_radps : UnitDelay  InitialCondition=w0  SampleTime=-1
  whlRadius : Gain  Gain=R  OutMin=0  OutMax=w_max/2
  Wheel Friction (N) : Outport
  Wheel Speed (rpm) : Outport  Port=2
  wires:
  M_abs_Nm/1 -> Subtract/1, Scope1/1
  v_mps/1 -> max_v_wr/1, v_wr/2
  w (rpm)/1 -> Wheel Speed (rpm)/1
  w_radps/1 -> Saturation/1
  Ts_over_Inertia/1 -> Sum/1
  Subtract/1 -> Ts_over_Inertia/1, Scope1/2
  Radius/1 -> Subtract/2
  Sign/1 -> Product/2
  max_v_wr/1 -> slip_ratio_percentage/2(max_v_wr)
  Product/1 -> Radius/1, Wheel Friction (N)/1
  v_wr/1 -> times100/1
  Abs/1 -> slip_ratio_percentage/1(abs_v_minus_wr)
  whlRadius/1 -> v_wr/1, max_v_wr/2
  slip_ratio_percentage/1(percent) -> friction_force_N/1, Slip Rate/1
  friction_force_N/1 -> Product/1
  Sum/1 -> w_radps/1
  Saturation/1 -> w (rpm)/1, whlRadius/1, Sum/2
  times100/1 -> Sign/1, Abs/1

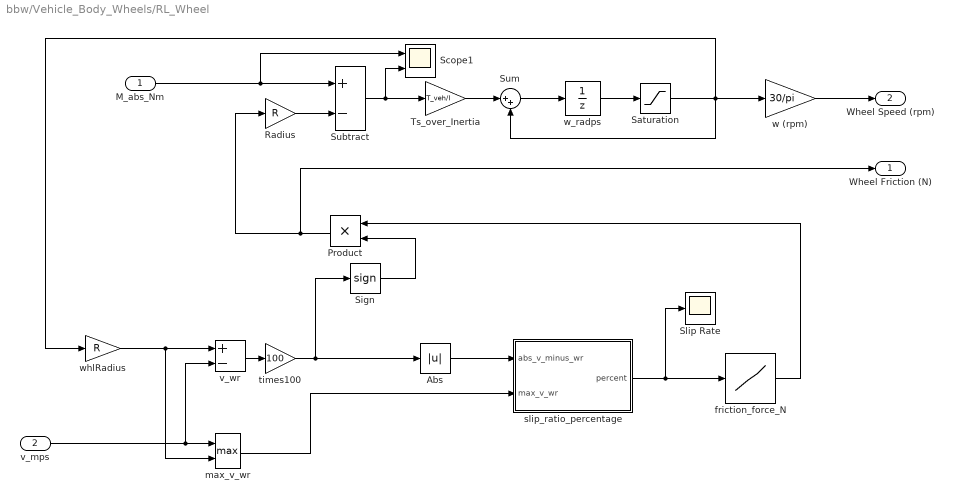
== system bbw/Vehicle_Body_Wheels/RL_Wheel ==
  M_abs_Nm : Inport
  v_mps : Inport  Port=2
  Abs : Abs
  Product : Product  RndMeth=Zero
  Radius : Gain  Gain=R
  Saturation : Saturate  UpperLimit=w_max  LowerLimit=0
  Scope1 : Scope  NumInputPorts=2
  Sign : Signum
  Slip Rate : Scope
  Subtract : Sum  Inputs=+-
  Sum : Sum  Inputs=|++
  Ts_over_Inertia : Gain  Gain=T_veh/I
  friction_force_N : Lookup  InputValues=Fc_table_x  Table=Fc_table_y  LookUpMeth=Interpolation-Use End Values  OutMin=0  OutMax=1000000  OutDataTypeStr=Inherit: Inherit via back propagation
  max_v_wr : MinMax  Function=max  Inputs=2
  slip_ratio_percentage : Subsystem
  times100 : Gain  Gain=100
  v_wr : Sum  Inputs=+-
  w (rpm) : Gain  Gain=30/pi  OutMin=0  OutMax=w_max*30/pi
  w_radps : UnitDelay  InitialCondition=w0  SampleTime=-1
  whlRadius : Gain  Gain=R  OutMin=0  OutMax=w_max/2
  Wheel Friction (N) : Outport
  Wheel Speed (rpm) : Outport  Port=2
  wires:
  M_abs_Nm/1 -> Subtract/1, Scope1/1
  v_mps/1 -> max_v_wr/1, v_wr/2
  w (rpm)/1 -> Wheel Speed (rpm)/1
  w_radps/1 -> Saturation/1
  Ts_over_Inertia/1 -> Sum/1
  Subtract/1 -> Ts_over_Inertia/1, Scope1/2
  Radius/1 -> Subtract/2
  Sign/1 -> Product/2
  max_v_wr/1 -> slip_ratio_percentage/2(max_v_wr)
  Product/1 -> Radius/1, Wheel Friction (N)/1
  v_wr/1 -> times100/1
  Abs/1 -> slip_ratio_percentage/1(abs_v_minus_wr)
  whlRadius/1 -> v_wr/1, max_v_wr/2
  slip_ratio_percentage/1(percent) -> friction_force_N/1, Slip Rate/1
  friction_force_N/1 -> Product/1
  Sum/1 -> w_radps/1
  Saturation/1 -> w (rpm)/1, whlRadius/1, Sum/2
  times100/1 -> Sign/1, Abs/1

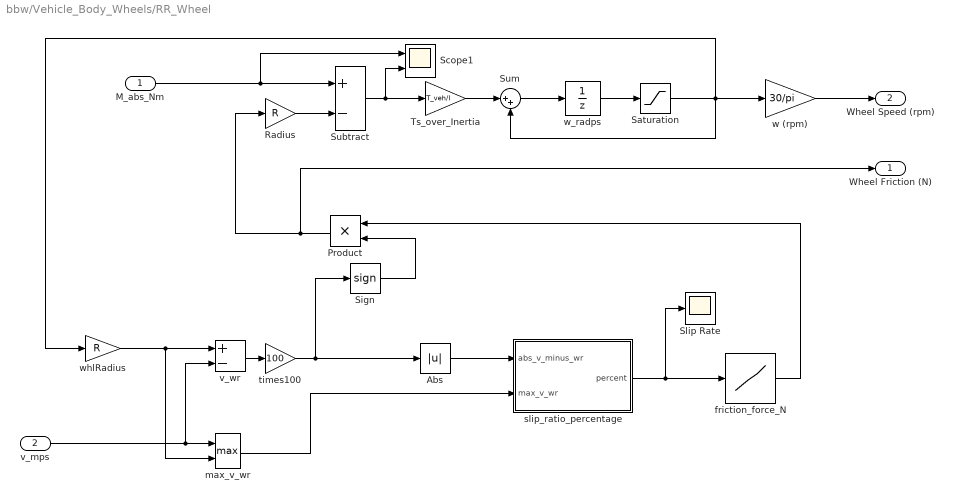
== system bbw/Vehicle_Body_Wheels/RR_Wheel ==
  M_abs_Nm : Inport
  v_mps : Inport  Port=2
  Abs : Abs
  Product : Product  RndMeth=Zero
  Radius : Gain  Gain=R
  Saturation : Saturate  UpperLimit=w_max  LowerLimit=0
  Scope1 : Scope  NumInputPorts=2
  Sign : Signum
  Slip Rate : Scope
  Subtract : Sum  Inputs=+-
  Sum : Sum  Inputs=|++
  Ts_over_Inertia : Gain  Gain=T_veh/I
  friction_force_N : Lookup  InputValues=Fc_table_x  Table=Fc_table_y  LookUpMeth=Interpolation-Use End Values  OutMin=0  OutMax=100000  OutDataTypeStr=Inherit: Inherit via back propagation
  max_v_wr : MinMax  Function=max  Inputs=2
  slip_ratio_percentage : Subsystem
  times100 : Gain  Gain=100
  v_wr : Sum  Inputs=+-
  w (rpm) : Gain  Gain=30/pi  OutMin=0  OutMax=w_max*30/pi
  w_radps : UnitDelay  InitialCondition=w0  SampleTime=-1
  whlRadius : Gain  Gain=R  OutMin=0  OutMax=w_max/2
  Wheel Friction (N) : Outport
  Wheel Speed (rpm) : Outport  Port=2
  wires:
  M_abs_Nm/1 -> Subtract/1, Scope1/1
  v_mps/1 -> max_v_wr/1, v_wr/2
  w (rpm)/1 -> Wheel Speed (rpm)/1
  w_radps/1 -> Saturation/1
  Ts_over_Inertia/1 -> Sum/1
  Subtract/1 -> Ts_over_Inertia/1, Scope1/2
  Radius/1 -> Subtract/2
  Sign/1 -> Product/2
  max_v_wr/1 -> slip_ratio_percentage/2(max_v_wr)
  Product/1 -> Radius/1, Wheel Friction (N)/1
  v_wr/1 -> times100/1
  Abs/1 -> slip_ratio_percentage/1(abs_v_minus_wr)
  whlRadius/1 -> v_wr/1, max_v_wr/2
  slip_ratio_percentage/1(percent) -> friction_force_N/1, Slip Rate/1
  friction_force_N/1 -> Product/1
  Sum/1 -> w_radps/1
  Saturation/1 -> w (rpm)/1, whlRadius/1, Sum/2
  times100/1 -> Sign/1, Abs/1

== system bbw/Vehicle_Body_Wheels/Vehicle Model ==
  Foce on RR Wheel : Inport
  Force on RL Wheel : Inport  Port=2
  Force on FR Wheel : Inport  Port=3
  Force on FL Wheel : Inport  Port=4
  Add : Sum  Inputs=++++
  Saturation : Saturate  UpperLimit=v_max  LowerLimit=0
  Sum : Sum  Inputs=|++
  Unit Delay : UnitDelay  InitialCondition=v0  SampleTime=-1
  sample_time_over_mass : Gain  Gain=T_veh/M
  Vehicle Speed (m/s) : Outport
  wires:
  sample_time_over_mass/1 -> Sum/1
  Add/1 -> sample_time_over_mass/1
  Force on FL Wheel/1 -> Add/4
  Force on FR Wheel/1 -> Add/3
  Force on RL Wheel/1 -> Add/2
  Foce on RR Wheel/1 -> Add/1
  Saturation/1 -> Vehicle Speed (m/s)/1, Sum/2
  Unit Delay/1 -> Saturation/1
  Sum/1 -> Unit Delay/1

== system bbw/Vehicle_Body_Wheels/FL_Wheel/slip_ratio_percentage ==
  abs_v_minus_wr : Inport
  max_v_wr : Inport  Port=2
  C_use_div : Constant  Value=use_division  SampleTime=-1
  C_zero : Constant  Value=0  SampleTime=-1
  Divide : Product  Inputs=*/
  Switch : Switch  Criteria=u2 > Threshold
  Switch1 : Switch  Criteria=u2 > Threshold
  binary_search_ratio : Stateflow chart  TreatAsAtomicUnit=on
  percent : Outport
  wires:
  max_v_wr/1 -> Switch/2, Divide/2, binary_search_ratio/2(max_v_wr)
  abs_v_minus_wr/1 -> Divide/1, binary_search_ratio/1(abs_v_minus_wr)
  Divide/1 -> Switch/1
  C_zero/1 -> Switch/3
  Switch/1 -> Switch1/1
  Switch1/1 -> percent/1
  C_use_div/1 -> Switch1/2
  binary_search_ratio/1(slip_ratio) -> Switch1/3

== system bbw/Vehicle_Body_Wheels/FR_Wheel/slip_ratio_percentage ==
  abs_v_minus_wr : Inport
  max_v_wr : Inport  Port=2
  C_use_div : Constant  Value=use_division  SampleTime=-1
  C_zero : Constant  Value=0  SampleTime=-1
  Divide : Product  Inputs=*/
  Switch : Switch  Criteria=u2 > Threshold
  Switch1 : Switch  Criteria=u2 > Threshold
  binary_search_ratio : Stateflow chart  TreatAsAtomicUnit=on
  percent : Outport
  wires:
  max_v_wr/1 -> Switch/2, Divide/2, binary_search_ratio/2(max_v_wr)
  abs_v_minus_wr/1 -> Divide/1, binary_search_ratio/1(abs_v_minus_wr)
  Divide/1 -> Switch/1
  C_zero/1 -> Switch/3
  Switch/1 -> Switch1/1
  Switch1/1 -> percent/1
  C_use_div/1 -> Switch1/2
  binary_search_ratio/1(slip_ratio) -> Switch1/3

== system bbw/Vehicle_Body_Wheels/RL_Wheel/slip_ratio_percentage ==
  abs_v_minus_wr : Inport
  max_v_wr : Inport  Port=2
  C_use_div : Constant  Value=use_division  SampleTime=-1
  C_zero : Constant  Value=0  SampleTime=-1
  Divide : Product  Inputs=*/
  Switch : Switch  Criteria=u2 > Threshold
  Switch1 : Switch  Criteria=u2 > Threshold
  binary_search_ratio : Stateflow chart  TreatAsAtomicUnit=on
  percent : Outport
  wires:
  max_v_wr/1 -> Switch/2, Divide/2, binary_search_ratio/2(max_v_wr)
  abs_v_minus_wr/1 -> Divide/1, binary_search_ratio/1(abs_v_minus_wr)
  Divide/1 -> Switch/1
  C_zero/1 -> Switch/3
  Switch/1 -> Switch1/1
  Switch1/1 -> percent/1
  C_use_div/1 -> Switch1/2
  binary_search_ratio/1(slip_ratio) -> Switch1/3

== system bbw/Vehicle_Body_Wheels/RR_Wheel/slip_ratio_percentage ==
  abs_v_minus_wr : Inport
  max_v_wr : Inport  Port=2
  C_use_div : Constant  Value=use_division  SampleTime=-1
  C_zero : Constant  Value=0  SampleTime=-1
  Divide : Product  Inputs=*/
  Switch : Switch  Criteria=u2 > Threshold
  Switch1 : Switch  Criteria=u2 > Threshold
  binary_search_ratio : Stateflow chart  TreatAsAtomicUnit=on
  percent : Outport
  wires:
  max_v_wr/1 -> Switch/2, Divide/2, binary_search_ratio/2(max_v_wr)
  abs_v_minus_wr/1 -> Divide/1, binary_search_ratio/1(abs_v_minus_wr)
  Divide/1 -> Switch/1
  C_zero/1 -> Switch/3
  Switch/1 -> Switch1/1
  Switch1/1 -> percent/1
  C_use_div/1 -> Switch1/2
  binary_search_ratio/1(slip_ratio) -> Switch1/3

== stateflow chart Vehicle_Body_Wheels/FL_Wheel/slip_ratio_percentage/binary_search_ratio ==
  (default) -> (junction 9) : /* check boundary conditions */
  (junction 9) -> (junction 10) [order 1] : [abs_v_minus_wr == 0 || max_v_wr == 0]
  (junction 9) -> (junction 11) [order 2]
  (junction 10) -> (junction 15) : {slip_ratio = 0;}
  (junction 11) -> (junction 12) [order 1] : [abs_v_minus_wr >= 100*max_v_wr]
  (junction 11) -> (junction 13) [order 2] : {idx_min = 0;
      | idx_max = 99;} /* start binary search */
  (junction 12) -> (junction 14) : {slip_ratio = 100;}
  (junction 13) -> (junction 14) [order 3] : {slip_ratio = 20;}
      | /* if idx_max < idx_min, return 20%. The case should never happen */
  (junction 14) -> (junction 15)
  (junction 20) -> (junction 13) : /* go back for iterative search */
  (junction 15) -> (junction 26) : /* terminate the flow */
  (junction 13) -> (junction 17) [order 1] : [idx_max == idx_min]
      | /* decide if idx_min is idx_max
      | or idx_max + 1 */
  (junction 13) -> (junction 16) [order 2] : [idx_max > idx_min]
  (junction 16) -> (junction 18) : {idx_mid = (idx_min + idx_max)/2;}
      | /* the middle index */
  (junction 17) -> (junction 23) : {idx_mid = idx_max;}
  (junction 18) -> (junction 19) [order 1] : [abs_v_minus_wr < idx_mid * max_v_wr]
      | /* if slip ratio is smaller than idx_mid */
  (junction 19) -> (junction 20) : {idx_max = idx_mid - 1;}
      | /* choose lower part */
  (junction 18) -> (junction 21) [order 2]
  (junction 22) -> (junction 20) : {idx_min = idx_mid +1;}
      | /* choose upper part */
  (junction 21) -> (junction 22) [order 1] : [abs_v_minus_wr > (idx_mid + 1)*max_v_wr]
      | /* if slip ratio is larger than idx_mid + 1 */
  (junction 21) -> (junction 23) [order 2]
  (junction 23) -> (junction 24) [order 1] : [abs_v_minus_wr - idx_mid * max_v_wr <= (idx_mid + 1)*max_v_wr - abs_v_minus_wr]
      | /* if slip ratio is closer to idx_mid than idx_mid + 1 */
  (junction 23) -> (junction 25) [order 2] : {slip_ratio = idx_mid + 1;}
  (junction 24) -> (junction 26) : {slip_ratio = idx_mid;}
  (junction 26) -> (junction 25) : /* terminate the flow */
  data: abs_v_minus_wr input double; max_v_wr input double; slip_ratio output double [0..100] =0; idx_mid local uint8 size=1 [0..99] =0; idx_min local uint8 size=1 [0..99] =0; idx_max local uint8 size=1 [0..99] =0

== stateflow chart Vehicle_Body_Wheels/FR_Wheel/slip_ratio_percentage/binary_search_ratio ==
  (default) -> (junction 60) : /* check boundary conditions */
  (junction 60) -> (junction 61) [order 1] : [abs_v_minus_wr == 0 || max_v_wr == 0]
  (junction 60) -> (junction 62) [order 2]
  (junction 61) -> (junction 66) : {slip_ratio = 0;}
  (junction 62) -> (junction 63) [order 1] : [abs_v_minus_wr >= 100*max_v_wr]
  (junction 62) -> (junction 64) [order 2] : {idx_min = 0;
      | idx_max = 99;} /* start binary search */
  (junction 63) -> (junction 65) : {slip_ratio = 100;}
  (junction 64) -> (junction 65) [order 3] : {slip_ratio = 20;}
      | /* if idx_max < idx_min, return 20%. The case should never happen */
  (junction 65) -> (junction 66)
  (junction 71) -> (junction 64) : /* go back for iterative search */
  (junction 66) -> (junction 77) : /* terminate the flow */
  (junction 64) -> (junction 68) [order 1] : [idx_max == idx_min]
      | /* decide if idx_min is idx_max
      | or idx_max + 1 */
  (junction 64) -> (junction 67) [order 2] : [idx_max > idx_min]
  (junction 67) -> (junction 69) : {idx_mid = (idx_min + idx_max)/2;}
      | /* the middle index */
  (junction 68) -> (junction 74) : {idx_mid = idx_max;}
  (junction 69) -> (junction 70) [order 1] : [abs_v_minus_wr < idx_mid * max_v_wr]
      | /* if slip ratio is smaller than idx_mid */
  (junction 70) -> (junction 71) : {idx_max = idx_mid - 1;}
      | /* choose lower part */
  (junction 69) -> (junction 72) [order 2]
  (junction 73) -> (junction 71) : {idx_min = idx_mid +1;}
      | /* choose upper part */
  (junction 72) -> (junction 73) [order 1] : [abs_v_minus_wr > (idx_mid + 1)*max_v_wr]
      | /* if slip ratio is larger than idx_mid + 1 */
  (junction 72) -> (junction 74) [order 2]
  (junction 74) -> (junction 75) [order 1] : [abs_v_minus_wr - idx_mid * max_v_wr <= (idx_mid + 1)*max_v_wr - abs_v_minus_wr]
      | /* if slip ratio is closer to idx_mid than idx_mid + 1 */
  (junction 74) -> (junction 76) [order 2] : {slip_ratio = idx_mid + 1;}
  (junction 75) -> (junction 77) : {slip_ratio = idx_mid;}
  (junction 77) -> (junction 76) : /* terminate the flow */
  data: abs_v_minus_wr input double; max_v_wr input double; slip_ratio output double [0..100] =0; idx_mid local uint8 size=1 [0..99] =0; idx_min local uint8 size=1 [0..99] =0; idx_max local uint8 size=1 [0..99] =0

== stateflow chart Vehicle_Body_Wheels/RL_Wheel/slip_ratio_percentage/binary_search_ratio ==
  (default) -> (junction 111) : /* check boundary conditions */
  (junction 111) -> (junction 112) [order 1] : [abs_v_minus_wr == 0 || max_v_wr == 0]
  (junction 111) -> (junction 113) [order 2]
  (junction 112) -> (junction 117) : {slip_ratio = 0;}
  (junction 113) -> (junction 114) [order 1] : [abs_v_minus_wr >= 100*max_v_wr]
  (junction 113) -> (junction 115) [order 2] : {idx_min = 0;
      | idx_max = 99;} /* start binary search */
  (junction 114) -> (junction 116) : {slip_ratio = 100;}
  (junction 115) -> (junction 116) [order 3] : {slip_ratio = 20;}
      | /* if idx_max < idx_min, return 20%. The case should never happen */
  (junction 116) -> (junction 117)
  (junction 122) -> (junction 115) : /* go back for iterative search */
  (junction 117) -> (junction 128) : /* terminate the flow */
  (junction 115) -> (junction 119) [order 1] : [idx_max == idx_min]
      | /* decide if idx_min is idx_max
      | or idx_max + 1 */
  (junction 115) -> (junction 118) [order 2] : [idx_max > idx_min]
  (junction 118) -> (junction 120) : {idx_mid = (idx_min + idx_max)/2;}
      | /* the middle index */
  (junction 119) -> (junction 125) : {idx_mid = idx_max;}
  (junction 120) -> (junction 121) [order 1] : [abs_v_minus_wr < idx_mid * max_v_wr]
      | /* if slip ratio is smaller than idx_mid */
  (junction 121) -> (junction 122) : {idx_max = idx_mid - 1;}
      | /* choose lower part */
  (junction 120) -> (junction 123) [order 2]
  (junction 124) -> (junction 122) : {idx_min = idx_mid +1;}
      | /* choose upper part */
  (junction 123) -> (junction 124) [order 1] : [abs_v_minus_wr > (idx_mid + 1)*max_v_wr]
      | /* if slip ratio is larger than idx_mid + 1 */
  (junction 123) -> (junction 125) [order 2]
  (junction 125) -> (junction 126) [order 1] : [abs_v_minus_wr - idx_mid * max_v_wr <= (idx_mid + 1)*max_v_wr - abs_v_minus_wr]
      | /* if slip ratio is closer to idx_mid than idx_mid + 1 */
  (junction 125) -> (junction 127) [order 2] : {slip_ratio = idx_mid + 1;}
  (junction 126) -> (junction 128) : {slip_ratio = idx_mid;}
  (junction 128) -> (junction 127) : /* terminate the flow */
  data: abs_v_minus_wr input double; max_v_wr input double; slip_ratio output double [0..100] =0; idx_mid local uint8 size=1 [0..99] =0; idx_min local uint8 size=1 [0..99] =0; idx_max local uint8 size=1 [0..99] =0

== stateflow chart Vehicle_Body_Wheels/RR_Wheel/slip_ratio_percentage/binary_search_ratio ==
  (default) -> (junction 162) : /* check boundary conditions */
  (junction 162) -> (junction 163) [order 1] : [abs_v_minus_wr == 0 || max_v_wr == 0]
  (junction 162) -> (junction 164) [order 2]
  (junction 163) -> (junction 168) : {slip_ratio = 0;}
  (junction 164) -> (junction 165) [order 1] : [abs_v_minus_wr >= 100*max_v_wr]
  (junction 164) -> (junction 166) [order 2] : {idx_min = 0;
      | idx_max = 99;} /* start binary search */
  (junction 165) -> (junction 167) : {slip_ratio = 100;}
  (junction 166) -> (junction 167) [order 3] : {slip_ratio = 20;}
      | /* if idx_max < idx_min, return 20%. The case should never happen */
  (junction 167) -> (junction 168)
  (junction 173) -> (junction 166) : /* go back for iterative search */
  (junction 168) -> (junction 179) : /* terminate the flow */
  (junction 166) -> (junction 170) [order 1] : [idx_max == idx_min]
      | /* decide if idx_min is idx_max
      | or idx_max + 1 */
  (junction 166) -> (junction 169) [order 2] : [idx_max > idx_min]
  (junction 169) -> (junction 171) : {idx_mid = (idx_min + idx_max)/2;}
      | /* the middle index */
  (junction 170) -> (junction 176) : {idx_mid = idx_max;}
  (junction 171) -> (junction 172) [order 1] : [abs_v_minus_wr < idx_mid * max_v_wr]
      | /* if slip ratio is smaller than idx_mid */
  (junction 172) -> (junction 173) : {idx_max = idx_mid - 1;}
      | /* choose lower part */
  (junction 171) -> (junction 174) [order 2]
  (junction 175) -> (junction 173) : {idx_min = idx_mid +1;}
      | /* choose upper part */
  (junction 174) -> (junction 175) [order 1] : [abs_v_minus_wr > (idx_mid + 1)*max_v_wr]
      | /* if slip ratio is larger than idx_mid + 1 */
  (junction 174) -> (junction 176) [order 2]
  (junction 176) -> (junction 177) [order 1] : [abs_v_minus_wr - idx_mid * max_v_wr <= (idx_mid + 1)*max_v_wr - abs_v_minus_wr]
      | /* if slip ratio is closer to idx_mid than idx_mid + 1 */
  (junction 176) -> (junction 178) [order 2] : {slip_ratio = idx_mid + 1;}
  (junction 177) -> (junction 179) : {slip_ratio = idx_mid;}
  (junction 179) -> (junction 178) : /* terminate the flow */
  data: abs_v_minus_wr input double; max_v_wr input double; slip_ratio output double [0..100] =0; idx_mid local uint8 size=1 [0..99] =0; idx_min local uint8 size=1 [0..99] =0; idx_max local uint8 size=1 [0..99] =0
